simulink model "testingExamples"  (R2019a)
settings: Solver=VariableStepAuto  StartTime=0.0  StopTime=stop_time/2  RelTol=1e-3
undefined symbols (not defined in the file or in its folder): mp, Ts
libraries: DSP_FPGA_Accelerated_Toolbox x2
settings Model: Creator=Bailey  LastModifiedBy=Bailey

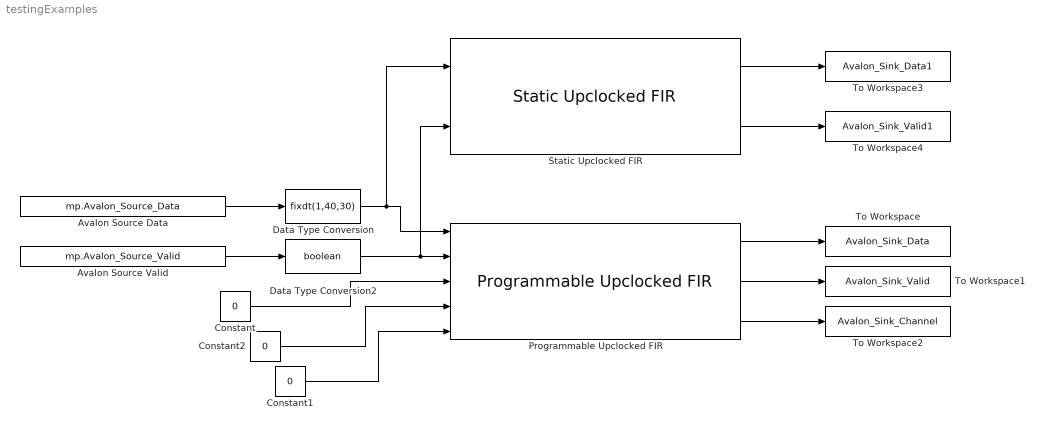
== system testingExamples ==
  "Avalon Source Data " : FromWorkspace  VariableName=mp.Avalon_Source_Data  OutDataTypeStr=double  SampleTime=mp.Ts_system
  Avalon Source Valid : FromWorkspace  VariableName=mp.Avalon_Source_Valid  OutDataTypeStr=double  SampleTime=mp.Ts_system
  Constant : Constant  Value=0  OutDataTypeStr=fixdt(1,34,29)  SampleTime=Ts
  Constant1 : Constant  Value=0  OutDataTypeStr=fixdt(0,2,0)  SampleTime=Ts*3
  Constant2 : Constant  Value=0  OutDataTypeStr=fixdt(0,3,0)  SampleTime=Ts*5
  Data Type Conversion : DataTypeConversion  OutDataTypeStr=fixdt(1,40,30)
  Data Type Conversion2 : DataTypeConversion  OutDataTypeStr=boolean
  Programmable Upclocked FIR : DSP_FPGA_Accelerated_Toolbox/Programmable Upclocked FIR  B_k=[0.5,0.5]  Ts=Ts  Ts_system=Ts_system  Added_Delay=0  W_bits=30  F_bits=20
  Static Upclocked FIR : DSP_FPGA_Accelerated_Toolbox/Static Upclocked FIR  B_k=[0.5,0.5]  Ts=Ts  Ts_system=Ts_system  Added_Delay=0  W_bits=30  F_bits=24
  To Workspace : ToWorkspace  VariableName=Avalon_Sink_Data  SaveFormat=Timeseries  SampleTime=-1
  To Workspace1 : ToWorkspace  VariableName=Avalon_Sink_Valid  SaveFormat=Timeseries  SampleTime=-1
  To Workspace2 : ToWorkspace  VariableName=Avalon_Sink_Channel  SaveFormat=Timeseries  SampleTime=-1
  To Workspace3 : ToWorkspace  VariableName=Avalon_Sink_Data1  SaveFormat=Timeseries  SampleTime=-1
  To Workspace4 : ToWorkspace  VariableName=Avalon_Sink_Valid1  SaveFormat=Timeseries  SampleTime=-1
  wires:
  Avalon Source Valid/1 -> Data Type Conversion2/1
  "Avalon Source Data "/1 -> Data Type Conversion/1
  Data Type Conversion/1 -> Static Upclocked FIR/1, Programmable Upclocked FIR/1
  Data Type Conversion2/1 -> Static Upclocked FIR/2, Programmable Upclocked FIR/2
  Constant/1 -> Programmable Upclocked FIR/3
  Programmable Upclocked FIR/1 -> To Workspace/1
  Programmable Upclocked FIR/2 -> To Workspace1/1
  Programmable Upclocked FIR/3 -> To Workspace2/1
  Constant1/1 -> Programmable Upclocked FIR/5
  Constant2/1 -> Programmable Upclocked FIR/4
  Static Upclocked FIR/2 -> To Workspace4/1
  Static Upclocked FIR/1 -> To Workspace3/1
